simulink model "EKF"  (R2021b)
settings: Solver=ode4  StartTime=0.0  StopTime=200  FixedStep=0.02  RelTol=1e-3
libraries: commchan3 x2
(part 4 of 4)

== matlab function EKF/Real System ==
  data: y input; xhat output; u input; Pcov output
function [xhat, Pcov]= fcn(y, u)
    Ts = 0.02;
    Qk = eye(5);
    Qk(1,1) = 1e-7;
    Qk(2,2) = 1e-7;
    Qk(3,3) = 1e-7;
    Qk(4,4) = 1e-5;
    Qk(5,5) = 1e-2;
    Rk = 1e-6;
    C = [0, 1, 0, 0, 0];
    
    persistent xhat_p Pcov_p;
    
    if isempty(xhat_p)
        xhat_p = [0;0;0;1/2;4];
        Pcov_p = 1000*ones(5, 5);
    end
    
    xkm = Fd(xhat_p, u, Ts);
    Fk = J_wrtX(xhat_p, u, Ts);
    Pkm = Fk*Pcov_p*Fk' + Qk;
    
    y_err = y - C*xkm;
    Sk = C*Pkm*C' + Rk;
    Kk = Pkm * C'*inv(Sk);
    xhat = xkm + Kk*y_err;
    Pcov_final = (eye(5) - Kk*C)*Pkm;
    
    Pcov = reshape(Pcov_final, [25, 1]);
    
    xhat_p = xhat;
    Pcov_p = Pcov_final;

    function X1 = Fd(x, u, Ts)
        x1 = x(1);
        x2 = x(2);
        x3 = x(3);
        M = x(4);
        D = x(5);
        X1 = [x1 + (Ts*(6*x2 + Ts*x3 + Ts*(x3 - (Ts*(5*M*u + (x2 + (Ts*x3)/2)*(100*M + 5*D*M) + 10*M*(x1 + (Ts*x2)/2) + (x3 - (Ts*(5*M*u + 10*M*x1 + x3*(D*M + 5) + x2*(100*M + 5*D*M)))/2)*(D*M + 5)))/2) + Ts*(x3 - (Ts*(5*M*u + 10*M*x1 + x3*(D*M + 5) + x2*(100*M + 5*D*M)))/2)))/6;
             x2 - (Ts*(Ts*(5*M*u + (x2 + (Ts*x3)/2)*(100*M + 5*D*M) + 10*M*(x1 + (Ts*x2)/2) + (x3 - (Ts*(5*M*u + 10*M*x1 + x3*(D*M + 5) + x2*(100*M + 5*D*M)))/2)*(D*M + 5)) - 6*x3 + Ts*((x2 + (Ts*(x3 - (Ts*(5*M*u + 10*M*x1 + x3*(D*M + 5) + x2*(100*M + 5*D*M)))/2))/2)*(100*M + 5*D*M) + 5*M*u + 10*M*(x1 + (Ts*(x2 + (Ts*x3)/2))/2) + (D*M + 5)*(x3 - (Ts*(5*M*u + (x2 + (Ts*x3)/2)*(100*M + 5*D*M) + 10*M*(x1 + (Ts*x2)/2) + (x3 - (Ts*(5*M*u + 10*M*x1 + x3*(D*M + 5) + x2*(100*M + 5*D*M)))/2)*(D*M + 5)))/2)) + Ts*(5*M*u + 10*M*x1 + x3*(D*M + 5) + x2*(100*M + 5*D*M))))/6;
             x3 - (Ts*(2*(x2 + (Ts*(x3 - (Ts*(5*M*u + 10*M*x1 + x3*(D*M + 5) + x2*(100*M + 5*D*M)))/2))/2)*(100*M + 5*D*M) + 30*M*u + 10*M*x1 + x3*(D*M + 5) + 20*M*(x1 + (Ts*(x2 + (Ts*x3)/2))/2) + 2*(x2 + (Ts*x3)/2)*(100*M + 5*D*M) + 2*(D*M + 5)*(x3 - (Ts*(5*M*u + (x2 + (Ts*x3)/2)*(100*M + 5*D*M) + 10*M*(x1 + (Ts*x2)/2) + (x3 - (Ts*(5*M*u + 10*M*x1 + x3*(D*M + 5) + x2*(100*M + 5*D*M)))/2)*(D*M + 5)))/2) + 20*M*(x1 + (Ts*x2)/2) + (x3 - Ts*((x2 + (Ts*(x3 - (Ts*(5*M*u + 10*M*x1 + x3*(D*M + 5) + x2*(100*M + 5*D*M)))/2))/2)*(100*M + 5*D*M) + 5*M*u + 10*M*(x1 + (Ts*(x2 + (Ts*x3)/2))/2) + (D*M + 5)*(x3 - (Ts*(5*M*u + (x2 + (Ts*x3)/2)*(100*M + 5*D*M) + 10*M*(x1 + (Ts*x2)/2) + (x3 - (Ts*(5*M*u + 10*M*x1 + x3*(D*M + 5) + x2*(100*M + 5*D*M)))/2)*(D*M + 5)))/2)))*(D*M + 5) + x2*(100*M + 5*D*M) + 2*(x3 - (Ts*(5*M*u + 10*M*x1 + x3*(D*M + 5) + x2*(100*M + 5*D*M)))/2)*(D*M + 5) + (x2 + Ts*(x3 - (Ts*(5*M*u + (x2 + (Ts*x3)/2)*(100*M + 5*D*M) + 10*M*(x1 + (Ts*x2)/2) + (x3 - (Ts*(5*M*u + 10*M*x1 + x3*(D*M + 5) + x2*(100*M + 5*D*M)))/2)*(D*M + 5)))/2))*(100*M + 5*D*M) + 10*M*(x1 + Ts*(x2 + (Ts*(x3 - (Ts*(5*M*u + 10*M*x1 + x3*(D*M + 5) + x2*(100*M + 5*D*M)))/2))/2))))/6;
             M;
             D];
    end

    function Ad = J_wrtX(x, u, Ts)
        x1 = x(1);
        x2 = x(2);
        x3 = x(3);
        M = x(4);
        D = x(5);
        Ad = [1 - (Ts*(5*M*Ts^2 + (Ts^2*(10*M - 5*M*Ts*(D*M + 5)))/2))/6,-(Ts*((Ts^2*(100*M + 5*D*M))/2 + (Ts^2*(100*M + 5*M*Ts + 5*D*M - (Ts*(D*M + 5)*(100*M + 5*D*M))/2))/2 - 6))/6, (Ts*(Ts - Ts*((Ts*(D*M + 5))/2 - 1) + Ts*((Ts*((D*M + 5)*((Ts*(D*M + 5))/2 - 1) - (Ts*(100*M + 5*D*M))/2))/2 + 1)))/6, -(Ts*((Ts^2*(5*u + 10*x1 + D*x3 + x2*(5*D + 100)))/2 + (Ts^2*(5*u + 10*x1 + 5*Ts*x2 + (5*D + 100)*(x2 + (Ts*x3)/2) + D*(x3 - (Ts*(5*M*u + 10*M*x1 + x3*(D*M + 5) + x2*(100*M + 5*D*M)))/2) - (Ts*(D*M + 5)*(5*u + 10*x1 + D*x3 + x2*(5*D + 100)))/2))/2))/6,-(Ts*((Ts^2*(5*M*(x2 + (Ts*x3)/2) + M*(x3 - (Ts*(5*M*u + 10*M*x1 + x3*(D*M + 5) + x2*(100*M + 5*D*M)))/2) - (Ts*(D*M + 5)*(5*M*x2 + M*x3))/2))/2 + (Ts^2*(5*M*x2 + M*x3))/2))/6;
            -(Ts*(10*M*Ts + Ts*(10*M - 5*M*Ts*(D*M + 5)) - Ts*((5*M*Ts^2*(100*M + 5*D*M))/2 - 10*M + (Ts*(D*M + 5)*(10*M - 5*M*Ts*(D*M + 5)))/2)))/6, 1 - (Ts*(Ts*(100*M + 5*D*M) + Ts*(100*M + 5*M*Ts + 5*D*M - (Ts*(D*M + 5)*(100*M + 5*D*M))/2) - Ts*(((Ts^2*(100*M + 5*D*M))/4 - 1)*(100*M + 5*D*M) - 5*M*Ts + (Ts*(D*M + 5)*(100*M + 5*M*Ts + 5*D*M - (Ts*(D*M + 5)*(100*M + 5*D*M))/2))/2)))/6,-(Ts*(Ts*(D*M + 5) + Ts*((5*M*Ts^2)/2 + ((Ts*((D*M + 5)*((Ts*(D*M + 5))/2 - 1) - (Ts*(100*M + 5*D*M))/2))/2 + 1)*(D*M + 5) - (Ts*((Ts*(D*M + 5))/2 - 1)*(100*M + 5*D*M))/2) - Ts*((D*M + 5)*((Ts*(D*M + 5))/2 - 1) - (Ts*(100*M + 5*D*M))/2) - 6))/6, -(Ts*(Ts*(5*u + 10*x1 + 5*Ts*x2 + (5*D + 100)*(x2 + (Ts*x3)/2) + D*(x3 - (Ts*(5*M*u + 10*M*x1 + x3*(D*M + 5) + x2*(100*M + 5*D*M)))/2) - (Ts*(D*M + 5)*(5*u + 10*x1 + D*x3 + x2*(5*D + 100)))/2) + Ts*(5*u + 10*x1 + (5*D + 100)*(x2 + (Ts*(x3 - (Ts*(5*M*u + 10*M*x1 + x3*(D*M + 5) + x2*(100*M + 5*D*M)))/2))/2) + D*(x3 - (Ts*(5*M*u + (x2 + (Ts*x3)/2)*(100*M + 5*D*M) + 10*M*(x1 + (Ts*x2)/2) + (x3 - (Ts*(5*M*u + 10*M*x1 + x3*(D*M + 5) + x2*(100*M + 5*D*M)))/2)*(D*M + 5)))/2) + 5*Ts*(x2 + (Ts*x3)/2) - (Ts^2*(100*M + 5*D*M)*(5*u + 10*x1 + D*x3 + x2*(5*D + 100)))/4 - (Ts*(D*M + 5)*(5*u + 10*x1 + 5*Ts*x2 + (5*D + 100)*(x2 + (Ts*x3)/2) + D*(x3 - (Ts*(5*M*u + 10*M*x1 + x3*(D*M + 5) + x2*(100*M + 5*D*M)))/2) - (Ts*(D*M + 5)*(5*u + 10*x1 + D*x3 + x2*(5*D + 100)))/2))/2) + Ts*(5*u + 10*x1 + D*x3 + x2*(5*D + 100))))/6,-(Ts*(Ts*(5*M*(x2 + (Ts*x3)/2) + M*(x3 - (Ts*(5*M*u + 10*M*x1 + x3*(D*M + 5) + x2*(100*M + 5*D*M)))/2) - (Ts*(D*M + 5)*(5*M*x2 + M*x3))/2) + Ts*(5*M*x2 + M*x3) + Ts*(5*M*(x2 + (Ts*(x3 - (Ts*(5*M*u + 10*M*x1 + x3*(D*M + 5) + x2*(100*M + 5*D*M)))/2))/2) + M*(x3 - (Ts*(5*M*u + (x2 + (Ts*x3)/2)*(100*M + 5*D*M) + 10*M*(x1 + (Ts*x2)/2) + (x3 - (Ts*(5*M*u + 10*M*x1 + x3*(D*M + 5) + x2*(100*M + 5*D*M)))/2)*(D*M + 5)))/2) - (Ts*(D*M + 5)*(5*M*(x2 + (Ts*x3)/2) + M*(x3 - (Ts*(5*M*u + 10*M*x1 + x3*(D*M + 5) + x2*(100*M + 5*D*M)))/2) - (Ts*(D*M + 5)*(5*M*x2 + M*x3))/2))/2 - (Ts^2*(5*M*x2 + M*x3)*(100*M + 5*D*M))/4)))/6;
            (Ts*(10*M*((5*M*Ts^3)/2 - 1) - 50*M + 10*M*Ts*(D*M + 5) + 5*M*Ts^2*(100*M + 5*D*M) + Ts*(D*M + 5)*(10*M - 5*M*Ts*(D*M + 5)) + (Ts^2*(10*M - 5*M*Ts*(D*M + 5))*(100*M + 5*D*M))/2 - Ts*(D*M + 5)*((5*M*Ts^2*(100*M + 5*D*M))/2 - 10*M + (Ts*(D*M + 5)*(10*M - 5*M*Ts*(D*M + 5)))/2)))/6, (Ts*(2*((Ts^2*(100*M + 5*D*M))/4 - 1)*(100*M + 5*D*M) - 20*M*Ts - 300*M + ((Ts^2*(100*M + 5*M*Ts + 5*D*M - (Ts*(D*M + 5)*(100*M + 5*D*M))/2))/2 - 1)*(100*M + 5*D*M) - 15*D*M + Ts*(D*M + 5)*(100*M + 5*D*M) + Ts*(D*M + 5)*(100*M + 5*M*Ts + 5*D*M - (Ts*(D*M + 5)*(100*M + 5*D*M))/2) - Ts*(D*M + 5)*(((Ts^2*(100*M + 5*D*M))/4 - 1)*(100*M + 5*D*M) - 5*M*Ts + (Ts*(D*M + 5)*(100*M + 5*M*Ts + 5*D*M - (Ts*(D*M + 5)*(100*M + 5*D*M))/2))/2) + 10*M*Ts*((Ts^2*(100*M + 5*D*M))/4 - 1)))/6, 1 - (Ts*(5*M*Ts^2 - 2*(D*M + 5)*((Ts*(D*M + 5))/2 - 1) - (D*M + 5)*(Ts*((5*M*Ts^2)/2 + ((Ts*((D*M + 5)*((Ts*(D*M + 5))/2 - 1) - (Ts*(100*M + 5*D*M))/2))/2 + 1)*(D*M + 5) - (Ts*((Ts*(D*M + 5))/2 - 1)*(100*M + 5*D*M))/2) - 1) + Ts*(100*M + 5*D*M) + 2*((Ts*((D*M + 5)*((Ts*(D*M + 5))/2 - 1) - (Ts*(100*M + 5*D*M))/2))/2 + 1)*(D*M + 5) + D*M - Ts*((Ts*(D*M + 5))/2 - 1)*(100*M + 5*D*M) - 5*M*Ts^2*((Ts*(D*M + 5))/2 - 1) + Ts*((Ts*((D*M + 5)*((Ts*(D*M + 5))/2 - 1) - (Ts*(100*M + 5*D*M))/2))/2 + 1)*(100*M + 5*D*M) + 5))/6, -(Ts*(30*u + 60*x1 + 2*(5*D + 100)*(x2 + (Ts*(x3 - (Ts*(5*M*u + 10*M*x1 + x3*(D*M + 5) + x2*(100*M + 5*D*M)))/2))/2) + D*x3 + 10*Ts*x2 + 2*(5*D + 100)*(x2 + (Ts*x3)/2) + 10*Ts*(x2 + (Ts*(x3 - (Ts*(5*M*u + 10*M*x1 + x3*(D*M + 5) + x2*(100*M + 5*D*M)))/2))/2) + 2*D*(x3 - (Ts*(5*M*u + (x2 + (Ts*x3)/2)*(100*M + 5*D*M) + 10*M*(x1 + (Ts*x2)/2) + (x3 - (Ts*(5*M*u + 10*M*x1 + x3*(D*M + 5) + x2*(100*M + 5*D*M)))/2)*(D*M + 5)))/2) + D*(x3 - Ts*((x2 + (Ts*(x3 - (Ts*(5*M*u + 10*M*x1 + x3*(D*M + 5) + x2*(100*M + 5*D*M)))/2))/2)*(100*M + 5*D*M) + 5*M*u + 10*M*(x1 + (Ts*(x2 + (Ts*x3)/2))/2) + (D*M + 5)*(x3 - (Ts*(5*M*u + (x2 + (Ts*x3)/2)*(100*M + 5*D*M) + 10*M*(x1 + (Ts*x2)/2) + (x3 - (Ts*(5*M*u + 10*M*x1 + x3*(D*M + 5) + x2*(100*M + 5*D*M)))/2)*(D*M + 5)))/2))) + 10*Ts*(x2 + (Ts*x3)/2) + 2*D*(x3 - (Ts*(5*M*u + 10*M*x1 + x3*(D*M + 5) + x2*(100*M + 5*D*M)))/2) + x2*(5*D + 100) + (5*D + 100)*(x2 + Ts*(x3 - (Ts*(5*M*u + (x2 + (Ts*x3)/2)*(100*M + 5*D*M) + 10*M*(x1 + (Ts*x2)/2) + (x3 - (Ts*(5*M*u + 10*M*x1 + x3*(D*M + 5) + x2*(100*M + 5*D*M)))/2)*(D*M + 5)))/2)) - Ts*(D*M + 5)*(5*u + 10*x1 + (5*D + 100)*(x2 + (Ts*(x3 - (Ts*(5*M*u + 10*M*x1 + x3*(D*M + 5) + x2*(100*M + 5*D*M)))/2))/2) + D*(x3 - (Ts*(5*M*u + (x2 + (Ts*x3)/2)*(100*M + 5*D*M) + 10*M*(x1 + (Ts*x2)/2) + (x3 - (Ts*(5*M*u + 10*M*x1 + x3*(D*M + 5) + x2*(100*M + 5*D*M)))/2)*(D*M + 5)))/2) + 5*Ts*(x2 + (Ts*x3)/2) - (Ts^2*(100*M + 5*D*M)*(5*u + 10*x1 + D*x3 + x2*(5*D + 100)))/4 - (Ts*(D*M + 5)*(5*u + 10*x1 + 5*Ts*x2 + (5*D + 100)*(x2 + (Ts*x3)/2) + D*(x3 - (Ts*(5*M*u + 10*M*x1 + x3*(D*M + 5) + x2*(100*M + 5*D*M)))/2) - (Ts*(D*M + 5)*(5*u + 10*x1 + D*x3 + x2*(5*D + 100)))/2))/2) - Ts*(D*M + 5)*(5*u + 10*x1 + D*x3 + x2*(5*D + 100)) - (Ts^2*(100*M + 5*D*M)*(5*u + 10*x1 + D*x3 + x2*(5*D + 100)))/2 - (5*M*Ts^3*(5*u + 10*x1 + D*x3 + x2*(5*D + 100)))/2 - Ts*(D*M + 5)*(5*u + 10*x1 + 5*Ts*x2 + (5*D + 100)*(x2 + (Ts*x3)/2) + D*(x3 - (Ts*(5*M*u + 10*M*x1 + x3*(D*M + 5) + x2*(100*M + 5*D*M)))/2) - (Ts*(D*M + 5)*(5*u + 10*x1 + D*x3 + x2*(5*D + 100)))/2) - (Ts^2*(100*M + 5*D*M)*(5*u + 10*x1 + 5*Ts*x2 + (5*D + 100)*(x2 + (Ts*x3)/2) + D*(x3 - (Ts*(5*M*u + 10*M*x1 + x3*(D*M + 5) + x2*(100*M + 5*D*M)))/2) - (Ts*(D*M + 5)*(5*u + 10*x1 + D*x3 + x2*(5*D + 100)))/2))/2))/6, -(Ts*(5*M*x2 + M*x3 + 5*M*(x2 + Ts*(x3 - (Ts*(5*M*u + (x2 + (Ts*x3)/2)*(100*M + 5*D*M) + 10*M*(x1 + (Ts*x2)/2) + (x3 - (Ts*(5*M*u + 10*M*x1 + x3*(D*M + 5) + x2*(100*M + 5*D*M)))/2)*(D*M + 5)))/2)) + 10*M*(x2 + (Ts*(x3 - (Ts*(5*M*u + 10*M*x1 + x3*(D*M + 5) + x2*(100*M + 5*D*M)))/2))/2) + 2*M*(x3 - (Ts*(5*M*u + (x2 + (Ts*x3)/2)*(100*M + 5*D*M) + 10*M*(x1 + (Ts*x2)/2) + (x3 - (Ts*(5*M*u + 10*M*x1 + x3*(D*M + 5) + x2*(100*M + 5*D*M)))/2)*(D*M + 5)))/2) + M*(x3 - Ts*((x2 + (Ts*(x3 - (Ts*(5*M*u + 10*M*x1 + x3*(D*M + 5) + x2*(100*M + 5*D*M)))/2))/2)*(100*M + 5*D*M) + 5*M*u + 10*M*(x1 + (Ts*(x2 + (Ts*x3)/2))/2) + (D*M + 5)*(x3 - (Ts*(5*M*u + (x2 + (Ts*x3)/2)*(100*M + 5*D*M) + 10*M*(x1 + (Ts*x2)/2) + (x3 - (Ts*(5*M*u + 10*M*x1 + x3*(D*M + 5) + x2*(100*M + 5*D*M)))/2)*(D*M + 5)))/2))) + 10*M*(x2 + (Ts*x3)/2) + 2*M*(x3 - (Ts*(5*M*u + 10*M*x1 + x3*(D*M + 5) + x2*(100*M + 5*D*M)))/2) - (5*M*Ts^3*(5*M*x2 + M*x3))/2 - Ts*(D*M + 5)*(5*M*(x2 + (Ts*x3)/2) + M*(x3 - (Ts*(5*M*u + 10*M*x1 + x3*(D*M + 5) + x2*(100*M + 5*D*M)))/2) - (Ts*(D*M + 5)*(5*M*x2 + M*x3))/2) - (Ts^2*(100*M + 5*D*M)*(5*M*(x2 + (Ts*x3)/2) + M*(x3 - (Ts*(5*M*u + 10*M*x1 + x3*(D*M + 5) + x2*(100*M + 5*D*M)))/2) - (Ts*(D*M + 5)*(5*M*x2 + M*x3))/2))/2 - Ts*(D*M + 5)*(5*M*x2 + M*x3) - (Ts^2*(5*M*x2 + M*x3)*(100*M + 5*D*M))/2 - Ts*(D*M + 5)*(5*M*(x2 + (Ts*(x3 - (Ts*(5*M*u + 10*M*x1 + x3*(D*M + 5) + x2*(100*M + 5*D*M)))/2))/2) + M*(x3 - (Ts*(5*M*u + (x2 + (Ts*x3)/2)*(100*M + 5*D*M) + 10*M*(x1 + (Ts*x2)/2) + (x3 - (Ts*(5*M*u + 10*M*x1 + x3*(D*M + 5) + x2*(100*M + 5*D*M)))/2)*(D*M + 5)))/2) - (Ts*(D*M + 5)*(5*M*(x2 + (Ts*x3)/2) + M*(x3 - (Ts*(5*M*u + 10*M*x1 + x3*(D*M + 5) + x2*(100*M + 5*D*M)))/2) - (Ts*(D*M + 5)*(5*M*x2 + M*x3))/2))/2 - (Ts^2*(5*M*x2 + M*x3)*(100*M + 5*D*M))/4)))/6;
            0,0, 0, 1,0;
            0,0, 0, 0,1];
    end
end

== matlab function EKF/State Space Equation ==
  data: x input; u input; dotx output
function dotx  = fcn(x, u)
D = 1.5;
M=4;
    Tg = 0.2;
    Rp = 0.05;
    Ki=2;
    dotx = zeros(3, 1);
    x1 = x(1);
    x2 = x(2);
    x3=x(3);
    dotx = [x2;x3;-Ki/(M*Tg)*x1-(D/(M*Tg)+1/(Rp*M*Tg))*x2-(D/M+1/Tg)*x3-1/(M*Tg)*u];

== matlab function EKF/MATLAB Function1 ==
  settings: updateMethod=DISCRETE
  data: y input; ymeas output
function ymeas = fcn(y)
    coder.extrinsic('gmdistribution');
    persistent gm;
    if isempty(gm)
        mu=[-0.1832;0.1601;-0.2891];
        sigma=cat(3,[0.0767],[0.0071],[0.0557]);
        w=[0.4719,0.3184,0.2097];
        gm=gmdistribution(mu,sigma,w);
    end
    noise = 0.0;
    noise = random(gm, 1);
    ymeas = y + 1e-3/0.2884*noise;
end
